simulink model "myexp5"  (R2022a)
settings: Solver=VariableStepAuto  StartTime=0.0  StopTime=100000  RelTol=1e-3
libraries: commrandsrc3 x3, commchan3 x3, commsink2 x3, dspswit3 x2, commblkcod2 x2
settings Model: Creator=惠普  LastModifiedBy=惠普

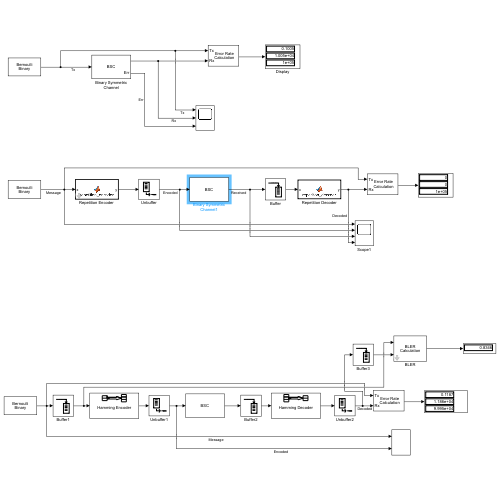
[thumbnail: Simulink's stored preview of the top-level diagram]
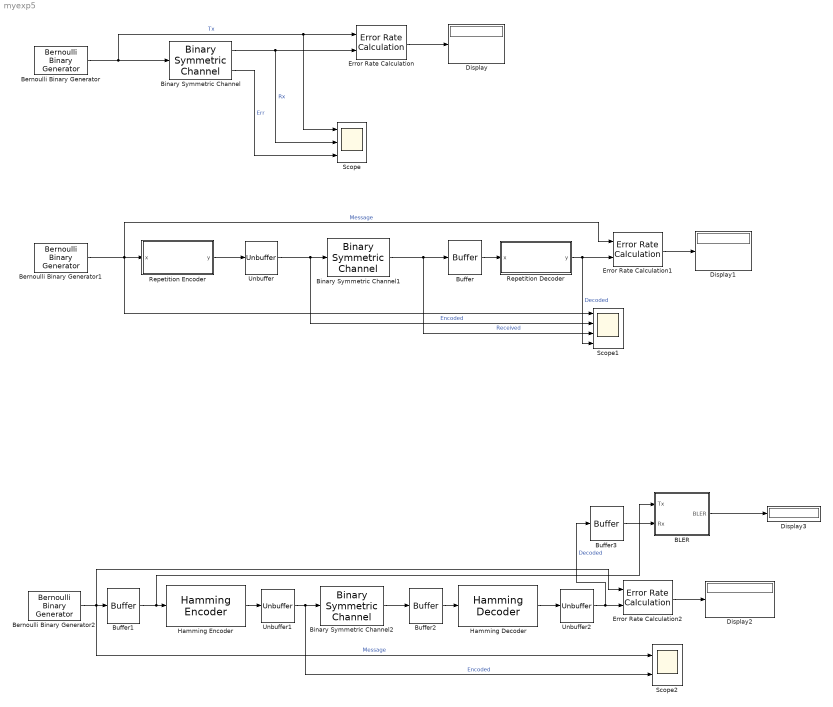
== system myexp5 ==
  BLER : Subsystem
      mask DialogControl ParameterGroupVar Prompt: 参数
      mask Display: disp(['BLER' char(10) 'Calculation']);
  Bernoulli Binary Generator : commrandsrc3/Bernoulli Binary Generator  ProbabilityOfZero=0.5  SeedSource=Auto  Seed=0  SampleTime=1  SamplesPerFrame=1  OutputDataType=double  SimulateUsing=Interpreted execution
  Bernoulli Binary Generator1 : commrandsrc3/Bernoulli Binary Generator  ProbabilityOfZero=0.5  SeedSource=Auto  Seed=0  SampleTime=1  SamplesPerFrame=1  OutputDataType=double  SimulateUsing=Interpreted execution
  Bernoulli Binary Generator2 : commrandsrc3/Bernoulli Binary Generator  ProbabilityOfZero=0.5  SeedSource=Auto  Seed=0  SampleTime=1  SamplesPerFrame=1  OutputDataType=double  SimulateUsing=Interpreted execution
  Binary Symmetric Channel : commchan3/Binary Symmetric Channel  ErrorProbability=0.1  ErrorVectorOutputPort=on  OutputDataType=double  OutputDataTypeSL=double  Seed=137  SimulateUsing=Code generation
      settings: SourceProductBaseCode=CM
  Binary Symmetric Channel1 : commchan3/Binary Symmetric Channel  ErrorProbability=0.003  ErrorVectorOutputPort=off  OutputDataType=double  OutputDataTypeSL=double  Seed=137  SimulateUsing=Code generation
      settings: SourceProductBaseCode=CM
  Binary Symmetric Channel2 : commchan3/Binary Symmetric Channel  ErrorProbability=0.1  ErrorVectorOutputPort=off  OutputDataType=double  OutputDataTypeSL=double  Seed=137  SimulateUsing=Code generation
      settings: SourceProductBaseCode=CM
  Buffer : Buffer  N=7  OutputFrames=off
  Buffer1 : Buffer  N=26  OutputFrames=off
  Buffer2 : Buffer  N=31  OutputFrames=off
  Buffer3 : Buffer  N=26  OutputFrames=off
  Display{,1..3} (4 alike) : Display
  Error Rate Calculation : commsink2/Error Rate Calculation  N=0  st_delay=0  cp_mode=Entire frame  subframe=[]  PMode=Port  WsName=ErrorVec  RsMode2=off  stop=off  numErr=100  maxBits=1e6
  Error Rate Calculation1 : commsink2/Error Rate Calculation  N=1  st_delay=0  cp_mode=Entire frame  subframe=[]  PMode=Port  WsName=ErrorVec  RsMode2=off  stop=off  numErr=100  maxBits=1e6
  Error Rate Calculation2 : commsink2/Error Rate Calculation  N=52  st_delay=0  cp_mode=Entire frame  subframe=[]  PMode=Port  WsName=ErrorVec  RsMode2=off  stop=off  numErr=100  maxBits=1e6
  Hamming Decoder : commblkcod2/Hamming Decoder  n=31  k=26
      settings: SourceProductBaseCode=CM
  Hamming Encoder : commblkcod2/Hamming Encoder  n=31  k=26
      settings: SourceProductBaseCode=CM
  Repetition Decoder : MATLAB Function  TreatAsAtomicUnit=on
  "Repetition Encoder " : MATLAB Function  TreatAsAtomicUnit=on  mask{n=7}
      mask prompts: n "number of repetitions"
  Scope : Scope  NumInputPorts=3
  Scope1 : Scope  NumInputPorts=4
  Scope2 : Scope  NumInputPorts=2
  Unbuffer : Unbuffer
  Unbuffer1 : Unbuffer
  Unbuffer2 : Unbuffer
  wires:
  Bernoulli Binary Generator/1 -> Scope/1, Error Rate Calculation/1, Binary Symmetric Channel/1  "Tx"
  Binary Symmetric Channel/1 -> Scope/2, Error Rate Calculation/2  "Rx"
  Binary Symmetric Channel/2 -> Scope/3  "Err"
  Error Rate Calculation/1 -> Display/1
  Bernoulli Binary Generator1/1 -> Error Rate Calculation1/1, Scope1/1, "Repetition Encoder "/1(x)  "Message"
  "Repetition Encoder "/1(y) -> Unbuffer/1
  Unbuffer/1 -> Scope1/2, Binary Symmetric Channel1/1  "Encoded"
  Binary Symmetric Channel1/1 -> Scope1/3, Buffer/1  "Received"
  Buffer/1 -> Repetition Decoder/1(x)
  Repetition Decoder/1(y) -> Scope1/4, Error Rate Calculation1/2  "Decoded"
  Error Rate Calculation1/1 -> Display1/1
  Hamming Encoder/1 -> Unbuffer1/1
  Binary Symmetric Channel2/1 -> Buffer2/1
  Buffer2/1 -> Hamming Decoder/1
  Hamming Decoder/1 -> Unbuffer2/1
  Error Rate Calculation2/1 -> Display2/1
  Unbuffer2/1 -> Buffer3/1, Error Rate Calculation2/2  "Decoded"
  Buffer1/1 -> BLER/1(Tx), Hamming Encoder/1
  Unbuffer1/1 -> Scope2/2, Binary Symmetric Channel2/1  "Encoded"
  Bernoulli Binary Generator2/1 -> Scope2/1, Error Rate Calculation2/1, Buffer1/1  "Message"
  Buffer3/1 -> BLER/2(Rx)
  BLER/1(BLER) -> Display3/1

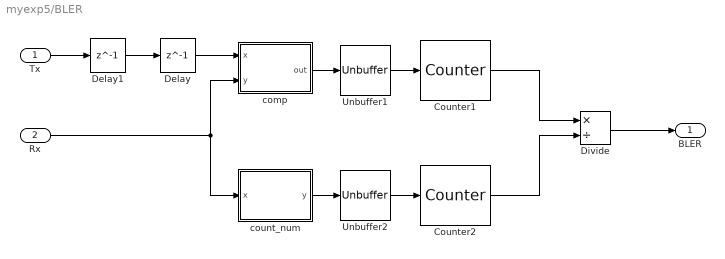
== system myexp5/BLER ==
  Tx : Inport
  Rx : Inport  Port=2
  Counter1 : dspswit3/Counter  Direction=Up  CountEvent=Rising edge  CounterSize=User defined  MaxCount=1000000  InitialCount=0  Output=Count  HitValue=32  ResetInput=off  SamplesPerFrame=1  Ts=1  CntDtype=double  HitDtype=Logical
  Counter2 : dspswit3/Counter  Direction=Up  CountEvent=Rising edge  CounterSize=User defined  MaxCount=1000000  InitialCount=0  Output=Count  HitValue=32  ResetInput=off  SamplesPerFrame=1  Ts=1  CntDtype=double  HitDtype=Logical
  Delay : Delay  DelayLength=1  InitialCondition=0
  Delay1 : Delay  DelayLength=1  InitialCondition=0
  Divide : Product  Inputs=*/
  Unbuffer1 : Unbuffer
  Unbuffer2 : Unbuffer
  comp : MATLAB Function  TreatAsAtomicUnit=on
  count_num : MATLAB Function  TreatAsAtomicUnit=on
  BLER : Outport
  wires:
  Rx/1 -> count_num/1(x), comp/2(y)
  Counter1/1 -> Divide/1
  Divide/1 -> BLER/1
  Counter2/1 -> Divide/2
  Tx/1 -> Delay1/1
  Delay1/1 -> Delay/1
  Delay/1 -> comp/1(x)
  Unbuffer1/1 -> Counter1/1
  comp/1(out) -> Unbuffer1/1
  count_num/1(y) -> Unbuffer2/1
  Unbuffer2/1 -> Counter2/1

== matlab function myexp5/Repetition Encoder  ==
  data: x input; y output; n parameter
function y = repetition_encoder(x, n)
y = repelem([x],n)';

== matlab function myexp5/BLER/comp ==
  data: x input; out output; y input
function out = comp(x,y)
len = length(x);
out = zeros(len,1);
for p = 1:len
    if (x(p) ~= y(p))
        out(1,1) = 1;
        return
    end
end
return

== matlab function myexp5/BLER/count_num ==
  data: x input; y output
function y = count_num(x)
len = length(x);
y = zeros(len,1);
y(1,1) = 1;
return

== matlab function myexp5/Repetition Decoder ==
  data: x input; y output
function y = repetition_decoder(x)
n0 = length(find(x == 0));
n1 = length(find(x == 1));
if(n0 >= n1)
    y = 0;
else
    y = 1;
end
